simulink model "test_model"  (R2019b)
settings: Solver=VariableStepAuto  StartTime=0.0  StopTime=10.0  RelTol=1e-3
libraries: simulink x2
settings Model: Creator=yafta  LastModifiedBy=yafta

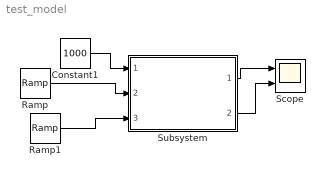
== system test_model ==
  Constant1 : Constant  Value=1000
  Ramp : simulink/Sources/Ramp  slope=0.02  start=0  InitialOutput=0
  Ramp1 : simulink/Sources/Ramp  slope=0.01  start=2  InitialOutput=0
  Scope : Scope  NumInputPorts=2
  Subsystem : Subsystem  ReferencedSubsystem=tire_model
  wires:
  Constant1/1 -> Subsystem/1
  Ramp/1 -> Subsystem/2
  Ramp1/1 -> Subsystem/3
  Subsystem/1 -> Scope/1
  Subsystem/2 -> Scope/2
